simulink model "PID_Controller_Tunning"  (R2022b)
settings: Solver=VariableStepAuto  StartTime=0.0  StopTime=30  RelTol=1e-3
settings Model: Creator=Mo_7atem  LastModifiedBy=Mo_7atem

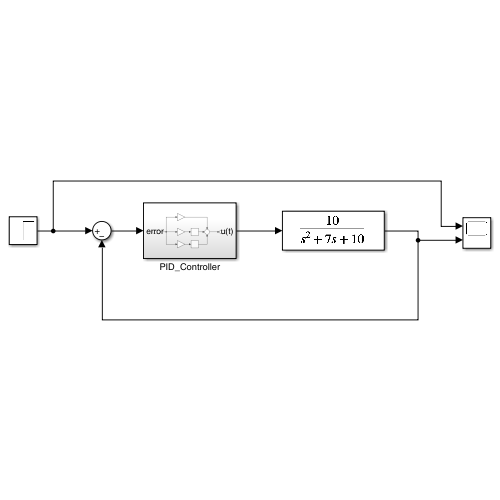
[thumbnail: Simulink's stored preview of the top-level diagram]
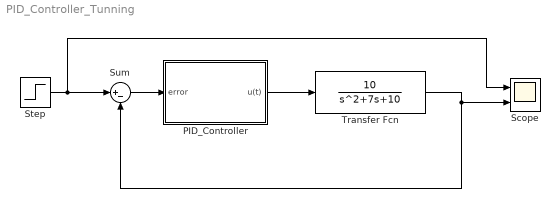
== system PID_Controller_Tunning ==
  PID_Controller : Subsystem
  Scope : Scope  NumInputPorts=2
  Step : Step  SampleTime=0
  Sum : Sum  Inputs=|+-
  Transfer Fcn : TransferFcn  Numerator=[10]  Denominator=[1 7 10]
  wires:
  Transfer Fcn/1 -> Sum/2, Scope/2
  Step/1 -> Scope/1, Sum/1
  PID_Controller/1(u(t)) -> Transfer Fcn/1
  Sum/1 -> PID_Controller/1(error)

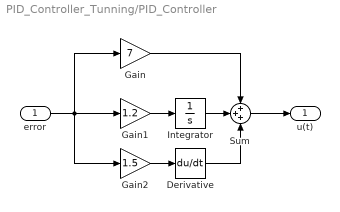
== system PID_Controller_Tunning/PID_Controller ==
  error : Inport
  Derivative : Derivative
  Gain : Gain  Gain=7
  Gain1 : Gain  Gain=1.2
  Gain2 : Gain  Gain=1.5
  Integrator : Integrator
  Sum : Sum  Inputs=+++
  u(t) : Outport
  wires:
  error/1 -> Gain2/1, Gain/1, Gain1/1
  Gain1/1 -> Integrator/1
  Integrator/1 -> Sum/2
  Gain/1 -> Sum/1
  Sum/1 -> u(t)/1
  Gain2/1 -> Derivative/1
  Derivative/1 -> Sum/3
